simulink model "model"  (R2024a)
settings: Solver=VariableStepAuto  StartTime=0.0  StopTime=250  RelTol=1e-8  AbsTol=1e-9
libraries: dspstat3 x4, simulink x1
settings Model: Creator=evgenijkondratev  LastModifiedBy=evgenijkondratev

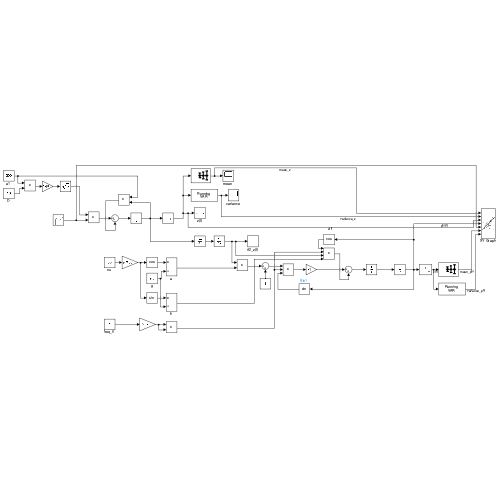
[thumbnail: Simulink's stored preview of the top-level diagram]
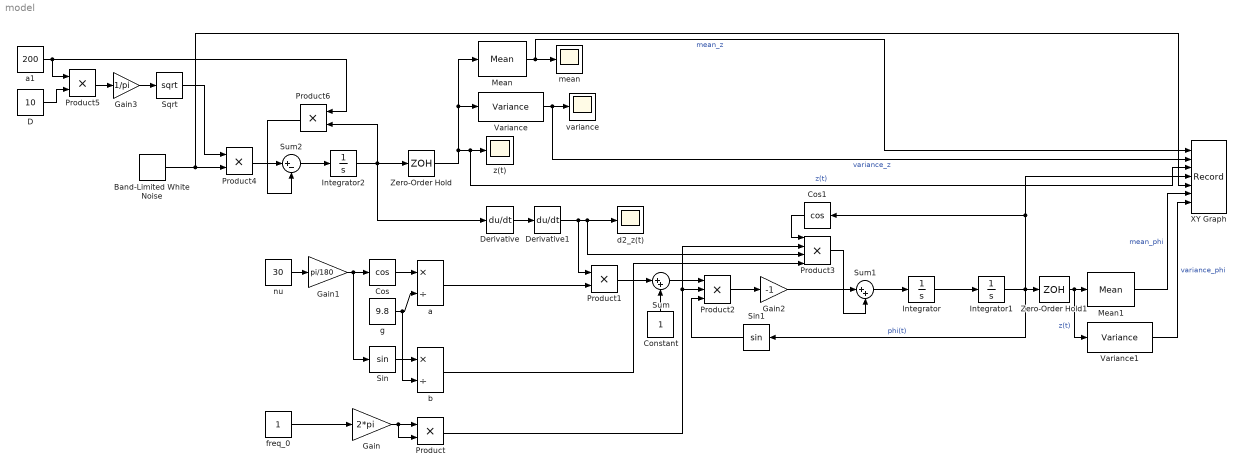
== system model ==
  Band-Limited White Noise : simulink/Sources/Band-Limited White Noise  Cov=[10]  Ts=0.001  seed=[23341]
  Constant : Constant
  Cos : Trigonometry  Operator=cos
  Cos1 : Trigonometry  Operator=cos
  D : Constant  Value=10
  Derivative : Derivative
  Derivative1 : Derivative
  Gain : Gain  Gain=2*pi
  Gain1 : Gain  Gain=pi/180
  Gain2 : Gain  Gain=-1
  Gain3 : Gain  Gain=1/pi
  Integrator : Integrator
  Integrator1 : Integrator
  Integrator2 : Integrator
  Mean : dspstat3/Mean  run=on  InputProcessing=Columns as channels (frame based)  reset_popup=None  directionMode=Each column  dimension=1  roiEnable=off  roiType=Rectangles  roiPortion=Entire ROI  roiOutput=Individual statistics for each ROI  roiFlag=off  roundingMode=Floor  overflowMode=off  outputDataTypeStr=Inherit: Same as accumulator  outputMin=[]  outputMax=[]  outputLastDataTypeStr=Inherit: Same as accumulator
  Mean1 : dspstat3/Mean  run=on  InputProcessing=Columns as channels (frame based)  reset_popup=None  directionMode=Each column  dimension=1  roiEnable=off  roiType=Rectangles  roiPortion=Entire ROI  roiOutput=Individual statistics for each ROI  roiFlag=off  roundingMode=Floor  overflowMode=off  outputDataTypeStr=Inherit: Same as accumulator  outputMin=[]  outputMax=[]  outputLastDataTypeStr=Inherit: Same as accumulator
  Product{,1,4..6} (5 alike) : Product
  Product2 : Product  Inputs=3
  Product3 : Product  Inputs=4
  Sin : Trigonometry
  Sin1 : Trigonometry
  Sqrt : Sqrt
  Sum : Sum  Inputs=|++
  Sum1 : Sum  Inputs=|++
  Sum2 : Sum  Inputs=|+-
  Variance : dspstat3/Variance  run=on  InputProcessing=Columns as channels (frame based)  reset_popup=None  directionMode=Each column  dimension=1  roiEnable=off  roiType=Rectangles  roiPortion=Entire ROI  roiOutput=Individual statistics for each ROI  roiFlag=off  roundingMode=Floor  overflowMode=off
  Variance1 : dspstat3/Variance  run=on  InputProcessing=Columns as channels (frame based)  reset_popup=None  directionMode=Each column  dimension=1  roiEnable=off  roiType=Rectangles  roiPortion=Entire ROI  roiOutput=Individual statistics for each ROI  roiFlag=off  roundingMode=Floor  overflowMode=off
  XY Graph : Record  FileSettingsInternal="{\"entries\":[{\"content\":{\"excelSettings\":{\"content\":{},\"type\":\"Streamout.ExcelSettings\"}},\"type\":\"Streamout.FileSettingStorage\",\"uuid\":\"\"}],\"packageUris\":[\"http:\\/\\/schema.mathworks.com\\/mf0\\/streamout_blocks\\/R2020a\"],\"version\":\"1.0\"}"  Layout=[1 1]  SignalsInternal="{\"entries\":[{\"content\":{\"signals\":[{\"content\":{\"blockPath\":[],\"dimensions\":[1],\"domain\":\"\",\"lineColor\":\"#a2142f\",\"plots\":[ 1 ],\"port\":1,\"sid\":[\"\"],\"signalID\":1,\"signalName\":\"mean_z\"},\"type\":\"RecordBlkView.Signal\",\"uuid\":\"\"},{\"content\":{\"blockPath\":[],\"dimensions\":[1],\"domain\":\"\",\"lineColor\":\"#139fff\",\"plots\":[ 1 ],\"port\":2,\"sid\":[\"\"],\"signalID\":2,\"signalName\":\"variance_z\"},\"type\":\"RecordBlkView.Signal\",\"uuid\":\"\"},{\"content\":{\"blockPath\":[],\"dimensions\":[1],\"domain\":\"\",\"lineColor\":\"#a2142f\",\"lineWidth\":2,\"port\":3,\"sid\":[\"\"],\"signalID\":3,\"signalName\":\"z(t)\"},\"type\":\"RecordBlkView.Signal\",\"uuid\":\"\"},{\"content\":{\"blockPath\":[],\"dimensions\":[1],\"domain\":\"\",\"lineColor\":\"#139fff\",\"lineWidth\":2,\"port\":4,\"sid\":[\"\"],\"signalID\":4,\"signalName\":\"phi(t)\"},\"type\":\"RecordBlkView.Signal\",\"uuid\":\"\"},{\"content\":{\"blockPath\":[],\"dimensions\":[1],\"domain\":\"\",\"lineColor\":\"#ff6929\",\"lineWidth\":2,\"port\":5,\"sid\":[\"\"],\"signalID\":5,\"signalName\":\"Band-Limited\\nWhite Noise\"},\"type\":\"RecordBlkView.Signal\",\"uuid\":\"\"},{\"content\":{\"blockPath\":[],\"dimensions\":[1],\"domain\":\"\",\"lineColor\":\"#b746ff\",\"lineWidth\":2,\"port\":6,\"sid\":[\"\"],\"signalID\":6,\"signalName\":\"mean_phi\"},\"type\":\"RecordBlkView.Signal\",\"uuid\":\"\"},{\"content\":{\"blockPath\":[],\"dimensions\":[1],\"domain\":\"\",\"lineColor\":\"#64d413\",\"lineWidth\":2,\"port\":7,\"sid\":[\"\"],\"signalID\":7,\"signalName\":\"variance_phi\"},\"type\":\"RecordBlkView.Signal\",\"uuid\":\"\"}]},\"type\":\"RecordBlkView.InputSignals\",\"uuid\":\"\"}],\"packageUris\":[\"http:\\/\\/schema.mathworks.com\\/mf0\\/streamout_blocks\\/R2020a\"],\"version\":\"1.0\"}"  VisualizationBindings="{\"xyplotplugin\":{\"info\":[{\"series\":[{\"bindingParametersList\":[{\"parameter\":\"X-Axis\",\"signalID\":1,\"signalName\":\"mean_z\"},{\"parameter\":\"Y-Axis\",\"signalID\":2,\"signalName\":\"variance_z\"}],\"seriesID\":0}],\"subplotID\":1}]}}"  CompatibilityTag=XY
  Zero-Order Hold : ZeroOrderHold  SampleTime=-1
  Zero-Order Hold1 : ZeroOrderHold  SampleTime=-1
  a : Product  Inputs=*/
  a1 : Constant  Value=200
  b : Product  Inputs=*/
  d2_z(t) : Scope
  freq_0 : Constant
  g : Constant  Value=9.8
  mean : Scope
  nu : Constant  Value=30
  variance : Scope
  z(t) : Scope
  wires:
  Mean/1 -> XY Graph/1, mean/1  "mean_z"
  Zero-Order Hold/1 -> Variance/1, Mean/1, XY Graph/3, z(t)/1  "z(t)"
  Variance/1 -> XY Graph/2, variance/1  "variance_z"
  Derivative/1 -> Derivative1/1
  Derivative1/1 -> Product1/1, Product3/3, d2_z(t)/1
  freq_0/1 -> Gain/1
  Gain/1 -> Product/2, Product/1
  nu/1 -> Gain1/1
  Gain1/1 -> Sin/1, Cos/1
  Cos/1 -> a/1
  g/1 -> b/2, a/2
  Sin/1 -> b/1
  a/1 -> Product1/2
  Product1/1 -> Sum/1
  Constant/1 -> Sum/2
  Sum/1 -> Product2/1
  Product/1 -> Product3/2, Product2/2
  Product2/1 -> Gain2/1
  b/1 -> Product3/4
  Gain2/1 -> Sum1/1
  Product3/1 -> Sum1/2
  Sum1/1 -> Integrator/1
  Integrator/1 -> Integrator1/1
  Integrator1/1 -> Zero-Order Hold1/1, XY Graph/4, Cos1/1, Sin1/1  "phi(t)"
  Mean1/1 -> XY Graph/6  "mean_phi"
  Variance1/1 -> XY Graph/7  "variance_phi"
  Zero-Order Hold1/1 -> Variance1/1, Mean1/1  "z(t)"
  Integrator2/1 -> Derivative/1, Zero-Order Hold/1, Product6/2
  Sum2/1 -> Integrator2/1
  a1/1 -> Product6/1, Product5/1
  D/1 -> Product5/2
  Sqrt/1 -> Product4/1
  Product6/1 -> Sum2/2
  Product4/1 -> Sum2/1
  Gain3/1 -> Sqrt/1
  Product5/1 -> Gain3/1
  Band-Limited White Noise/1 -> XY Graph/5, Product4/2
  Cos1/1 -> Product3/1
  Sin1/1 -> Product2/3
